simulink model "PresentationDiagram"  (R2020b)
settings: Solver=VariableStepAuto  StartTime=0.0  StopTime=10.0  RelTol=1e-3
model workspace (MAT data in the model file):
  kd = Simulink.Parameter
  kd.DataType = 'auto'
  kd.Dimensions = [0 0]
  ki = Simulink.Parameter
  ki.DataType = 'auto'
  ki.Dimensions = [0 0]
  kp = Simulink.Parameter
  kp.DataType = 'auto'
  kp.Dimensions = [0 0]
  ks = Simulink.Parameter
  ks.DataType = 'auto'
  ks.Dimensions = [0 0]
settings Model: Creator=barko  LastModifiedBy=barko

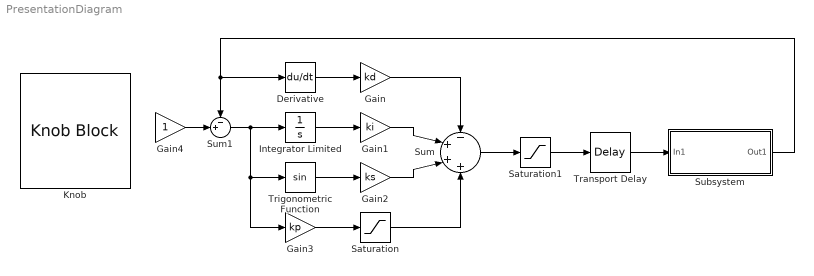
== system PresentationDiagram ==
  Derivative : Derivative
  Gain : Gain  Gain=kd
  Gain1 : Gain  Gain=ki
  Gain2 : Gain  Gain=ks
  Gain3 : Gain  Gain=kp
  Gain4 : Gain
  Integrator Limited : Integrator  LimitOutput=on  UpperSaturationLimit=0.2  LowerSaturationLimit=-0.2
  Knob : KnobBlock  LabelPosition=Hide  ScaleMax=180
  Saturation : Saturate
  Saturation1 : Saturate
  Subsystem : Subsystem
  Sum : Sum  Inputs=-|+|+|+
  Sum1 : Sum  Inputs=-+|
  Transport Delay : TransportDelay
  Trigonometric Function : Trigonometry
  wires:
  Trigonometric Function/1 -> Gain2/1
  Integrator Limited/1 -> Gain1/1
  Derivative/1 -> Gain/1
  Gain3/1 -> Saturation/1
  Saturation/1 -> Sum/4
  Gain2/1 -> Sum/3
  Gain1/1 -> Sum/2
  Gain/1 -> Sum/1
  Sum/1 -> Saturation1/1
  Saturation1/1 -> Transport Delay/1
  Sum1/1 -> Gain3/1, Trigonometric Function/1, Integrator Limited/1
  Gain4/1 -> Sum1/2
  Transport Delay/1 -> Subsystem/1(In1)
  Subsystem/1(Out1) -> Derivative/1, Sum1/1

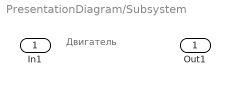
== system PresentationDiagram/Subsystem ==
  note: Двигатель
  In1 : Inport
  Out1 : Outport
